simulink model "complex_dbe_core"  (Simulink 7.1)
settings: Solver=ode45  StartTime=0.0  StopTime=1000  RelTol=1e-3
libraries: xbsIndex_r4 x308, cfa_library x64, casper_library_misc x6, simulink x2
(part 1 of 6)
settings Model: Creator=Administrator  LastModifiedBy=Administrator

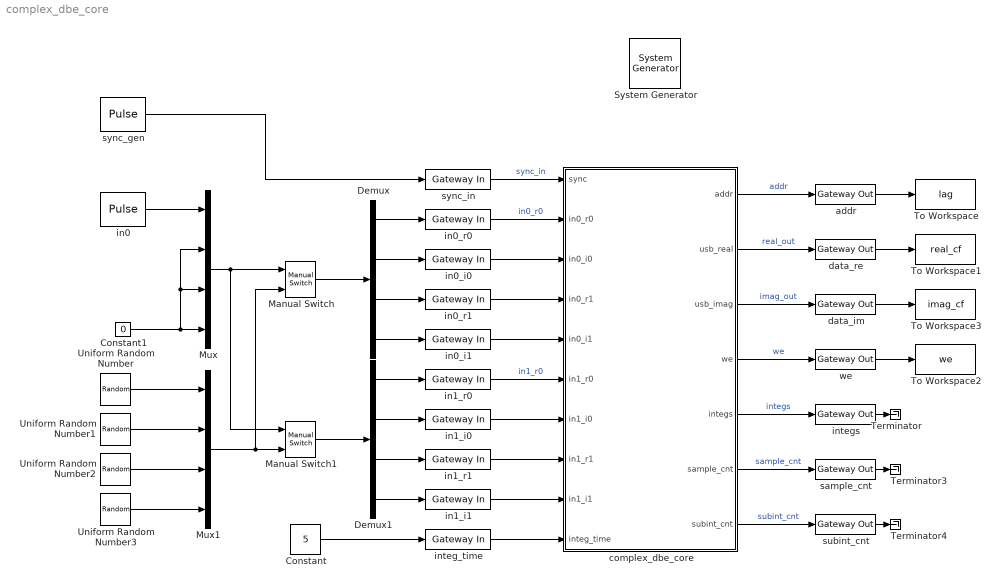
== system complex_dbe_core ==
  " System Generator" : xbsIndex_r4/ System Generator  Tag=genX  SystemSampleTime=-1  xilinxfamily=virtex2p  part=xc2vp50  speed=-7  package=ff1152  synthesis_tool=XST  clock_wrapper=Clock Enables  directory=./complex_dbe_core  testbench=off  simulink_period=1  sysclk_period=10  dcm_input_clock_period=100  incr_netlist=off  trim_vbits=Everywhere in SubSystem  dbl_ovrd=According to Block Masks  core_generation=According to Block Masks  run_coregen=off  deprecated_control=off  eval_field=0  block_type=sysgen
      settings: block_version=10.1.3
  Constant : Constant  Value=5  OutDataType=sfix(16)  OutScaling=2^0
  Constant1 : Constant  Value=0
  Demux : Demux
  Demux1 : Demux
  Manual Switch : simulink/Signal Routing/Manual Switch  SystemSampleTime=-1  sw=0  action=0  varsize=off
  Manual Switch1 : simulink/Signal Routing/Manual Switch  SystemSampleTime=-1  sw=0  action=0  varsize=off
  Mux : Mux
  Mux1 : Mux
  Terminator : Terminator
  Terminator3 : Terminator
  Terminator4 : Terminator
  To Workspace : ToWorkspace  VariableName=lag  SampleTime=-1  SaveFormat=Array
  To Workspace1 : ToWorkspace  VariableName=real_cf  SampleTime=-1  SaveFormat=Array
  To Workspace2 : ToWorkspace  VariableName=we  SampleTime=-1  SaveFormat=Array
  To Workspace3 : ToWorkspace  VariableName=imag_cf  SampleTime=-1  SaveFormat=Array
  Uniform Random Number : UniformRandomNumber  Minimum=0  Maximum=3  Seed=1111  SampleTime=1
  Uniform Random Number1 : UniformRandomNumber  Minimum=0  Maximum=3  Seed=2222  SampleTime=1
  Uniform Random Number2 : UniformRandomNumber  Minimum=0  Maximum=3  Seed=3333  SampleTime=1
  Uniform Random Number3 : UniformRandomNumber  Minimum=0  Maximum=3  Seed=4444  SampleTime=1
  addr : xbsIndex_r4/Gateway Out  hdl_port=on  timing_constraint=None  locs_specified=off  LOCs={}  block_type=gatewayout
      settings: infoedit="Gateway out block.  Converts Xilinx fixed point inputs into ouputs of type Simulink integer, double, or fixed point.<P><P>Hardware notes:  In hardware these blocks become top level output ports or are discarded, depending on how they are configured."  block_version=10.1.3
  complex_dbe_core : Subsystem
  data_im : xbsIndex_r4/Gateway Out  hdl_port=on  timing_constraint=None  locs_specified=off  LOCs={}  block_type=gatewayout
      settings: infoedit="Gateway out block.  Converts Xilinx fixed point inputs into ouputs of type Simulink integer, double, or fixed point.<P><P>Hardware notes:  In hardware these blocks become top level output ports or are discarded, depending on how they are configured."  block_version=10.1.3
  data_re : xbsIndex_r4/Gateway Out  hdl_port=on  timing_constraint=None  locs_specified=off  LOCs={}  block_type=gatewayout
      settings: infoedit="Gateway out block.  Converts Xilinx fixed point inputs into ouputs of type Simulink integer, double, or fixed point.<P><P>Hardware notes:  In hardware these blocks become top level output ports or are discarded, depending on how they are configured."  block_version=10.1.3
  in0 : DiscretePulseGenerator  Period=1e4  PhaseDelay=256+10+1+16*2
      settings: AttributesFormatString=%<PulseWidth> wide\npulse at %<PhaseDelay>\nevery %<Period>
  in0_i0 : xbsIndex_r4/Gateway In  arith_type=Unsigned  n_bits=2  bin_pt=0  quantization=Truncate  overflow=Wrap  period=1  dbl_ovrd=off  timing_constraint=None  locs_specified=off  LOCs={}  block_type=gatewayin
      settings: infoedit="Gateway in block.  Converts inputs of type Simulink integer, double and fixed point to  Xilinx fixed point type.<br><br>Hardware notes:  In hardware these blocks become top level input ports."  block_version=10.1.3
  in0_i1 : xbsIndex_r4/Gateway In  arith_type=Unsigned  n_bits=2  bin_pt=0  quantization=Truncate  overflow=Wrap  period=1  dbl_ovrd=off  timing_constraint=None  locs_specified=off  LOCs={}  block_type=gatewayin
      settings: infoedit="Gateway in block.  Converts inputs of type Simulink integer, double and fixed point to  Xilinx fixed point type.<br><br>Hardware notes:  In hardware these blocks become top level input ports."  block_version=10.1.3
  in0_r0 : xbsIndex_r4/Gateway In  arith_type=Unsigned  n_bits=2  bin_pt=0  quantization=Truncate  overflow=Flag as error  period=1  dbl_ovrd=off  timing_constraint=None  locs_specified=off  LOCs={}  block_type=gatewayin
      settings: infoedit="Gateway in block.  Converts inputs of type Simulink integer, double and fixed point to  Xilinx fixed point type.<br><br>Hardware notes:  In hardware these blocks become top level input ports."  block_version=10.1.3
  in0_r1 : xbsIndex_r4/Gateway In  arith_type=Unsigned  n_bits=2  bin_pt=0  quantization=Truncate  overflow=Wrap  period=1  dbl_ovrd=off  timing_constraint=None  locs_specified=off  LOCs={}  block_type=gatewayin
      settings: infoedit="Gateway in block.  Converts inputs of type Simulink integer, double and fixed point to  Xilinx fixed point type.<br><br>Hardware notes:  In hardware these blocks become top level input ports."  block_version=10.1.3
  in1_i0 : xbsIndex_r4/Gateway In  arith_type=Unsigned  n_bits=2  bin_pt=0  quantization=Truncate  overflow=Wrap  period=1  dbl_ovrd=off  timing_constraint=None  locs_specified=off  LOCs={}  block_type=gatewayin
      settings: infoedit="Gateway in block.  Converts inputs of type Simulink integer, double and fixed point to  Xilinx fixed point type.<br><br>Hardware notes:  In hardware these blocks become top level input ports."  block_version=10.1.3
  in1_i1 : xbsIndex_r4/Gateway In  arith_type=Unsigned  n_bits=2  bin_pt=0  quantization=Truncate  overflow=Wrap  period=1  dbl_ovrd=off  timing_constraint=None  locs_specified=off  LOCs={}  block_type=gatewayin
      settings: infoedit="Gateway in block.  Converts inputs of type Simulink integer, double and fixed point to  Xilinx fixed point type.<br><br>Hardware notes:  In hardware these blocks become top level input ports."  block_version=10.1.3
  in1_r0 : xbsIndex_r4/Gateway In  arith_type=Unsigned  n_bits=2  bin_pt=0  quantization=Truncate  overflow=Wrap  period=1  dbl_ovrd=off  timing_constraint=None  locs_specified=off  LOCs={}  block_type=gatewayin
      settings: infoedit="Gateway in block.  Converts inputs of type Simulink integer, double and fixed point to  Xilinx fixed point type.<br><br>Hardware notes:  In hardware these blocks become top level input ports."  block_version=10.1.3
  in1_r1 : xbsIndex_r4/Gateway In  arith_type=Unsigned  n_bits=2  bin_pt=0  quantization=Truncate  overflow=Wrap  period=1  dbl_ovrd=off  timing_constraint=None  locs_specified=off  LOCs={}  block_type=gatewayin
      settings: infoedit="Gateway in block.  Converts inputs of type Simulink integer, double and fixed point to  Xilinx fixed point type.<br><br>Hardware notes:  In hardware these blocks become top level input ports."  block_version=10.1.3
  integ_time : xbsIndex_r4/Gateway In  arith_type=Unsigned  n_bits=32  bin_pt=0  quantization=Truncate  overflow=Wrap  period=1  dbl_ovrd=off  timing_constraint=None  locs_specified=off  LOCs={}  block_type=gatewayin
      settings: infoedit="Gateway in block.  Converts inputs of type Simulink integer, double and fixed point to  Xilinx fixed point type.<P><P>Hardware notes:  In hardware these blocks become top level input ports."  block_version=10.1.3
  integs : xbsIndex_r4/Gateway Out  hdl_port=on  timing_constraint=None  locs_specified=off  LOCs={}  block_type=gatewayout
      settings: infoedit="Gateway out block.  Converts Xilinx fixed point inputs into ouputs of type Simulink integer, double, or fixed point.<P><P>Hardware notes:  In hardware these blocks become top level output ports or are discarded, depending on how they are configured."  block_version=10.1.3
  sample_cnt : xbsIndex_r4/Gateway Out  hdl_port=on  timing_constraint=None  locs_specified=off  LOCs={}  block_type=gatewayout
      settings: infoedit="Gateway out block.  Converts Xilinx fixed point inputs into ouputs of type Simulink integer, double, or fixed point.<P><P>Hardware notes:  In hardware these blocks become top level output ports or are discarded, depending on how they are configured."  block_version=10.1.3
  subint_cnt : xbsIndex_r4/Gateway Out  hdl_port=on  timing_constraint=None  locs_specified=off  LOCs={}  block_type=gatewayout
      settings: infoedit="Gateway out block.  Converts Xilinx fixed point inputs into ouputs of type Simulink integer, double, or fixed point.<P><P>Hardware notes:  In hardware these blocks become top level output ports or are discarded, depending on how they are configured."  block_version=10.1.3
  sync_gen : DiscretePulseGenerator  Period=32  PhaseDelay=10
      settings: AttributesFormatString=%<PulseWidth> wide\npulse at %<PhaseDelay>\nevery %<Period>
  sync_in : xbsIndex_r4/Gateway In  arith_type=Boolean  n_bits=16  bin_pt=14  quantization="Round  (unbiased: +/- Inf)"  overflow=Saturate  period=1  dbl_ovrd=off  timing_constraint=None  locs_specified=off  LOCs={}  block_type=gatewayin
      settings: infoedit="Gateway in block.  Converts inputs of type Simulink integer, double and fixed point to  Xilinx fixed point type.<P><P>Hardware notes:  In hardware these blocks become top level input ports."  block_version=10.1.3
  we : xbsIndex_r4/Gateway Out  hdl_port=on  timing_constraint=None  locs_specified=off  LOCs={}  block_type=gatewayout
      settings: infoedit="Gateway out block.  Converts Xilinx fixed point inputs into ouputs of type Simulink integer, double, or fixed point.<P><P>Hardware notes:  In hardware these blocks become top level output ports or are discarded, depending on how they are configured."  block_version=10.1.3
  wires:
  sync_in/1 -> complex_dbe_core/1(sync)  "sync_in"
  in0_r0/1 -> complex_dbe_core/2(in0_r0)  "in0_r0"
  in0_i0/1 -> complex_dbe_core/3(in0_i0)
  in0_r1/1 -> complex_dbe_core/4(in0_r1)
  in0_i1/1 -> complex_dbe_core/5(in0_i1)
  in1_r0/1 -> complex_dbe_core/6(in1_r0)  "in1_r0"
  in1_i0/1 -> complex_dbe_core/7(in1_i0)
  in1_r1/1 -> complex_dbe_core/8(in1_r1)
  in1_i1/1 -> complex_dbe_core/9(in1_i1)
  sync_gen/1 -> sync_in/1
  integ_time/1 -> complex_dbe_core/10(integ_time)
  Constant/1 -> integ_time/1
  addr/1 -> To Workspace/1
  data_re/1 -> To Workspace1/1
  we/1 -> To Workspace2/1
  complex_dbe_core/1(addr) -> addr/1  "addr"
  complex_dbe_core/2(usb_real) -> data_re/1  "real_out"
  data_im/1 -> To Workspace3/1
  complex_dbe_core/3(usb_imag) -> data_im/1  "imag_out"
  complex_dbe_core/4(we) -> we/1  "we"
  complex_dbe_core/5(integs) -> integs/1  "integs"
  integs/1 -> Terminator/1
  complex_dbe_core/6(sample_cnt) -> sample_cnt/1  "sample_cnt"
  sample_cnt/1 -> Terminator3/1
  complex_dbe_core/7(subint_cnt) -> subint_cnt/1  "subint_cnt"
  subint_cnt/1 -> Terminator4/1
  Demux/1 -> in0_r0/1
  Demux/2 -> in0_i0/1
  Demux/3 -> in0_r1/1
  Demux/4 -> in0_i1/1
  in0/1 -> Mux/1
  Constant1/1 -> Mux/4, Mux/2, Mux/3
  Demux1/1 -> in1_r0/1
  Demux1/2 -> in1_i0/1
  Demux1/3 -> in1_r1/1
  Demux1/4 -> in1_i1/1
  Uniform Random Number/1 -> Mux1/1
  Uniform Random Number1/1 -> Mux1/2
  Uniform Random Number2/1 -> Mux1/3
  Uniform Random Number3/1 -> Mux1/4
  Manual Switch/1 -> Demux/1
  Mux/1 -> Manual Switch/1, Manual Switch1/1
  Manual Switch1/1 -> Demux1/1
  Mux1/1 -> Manual Switch1/2, Manual Switch/2

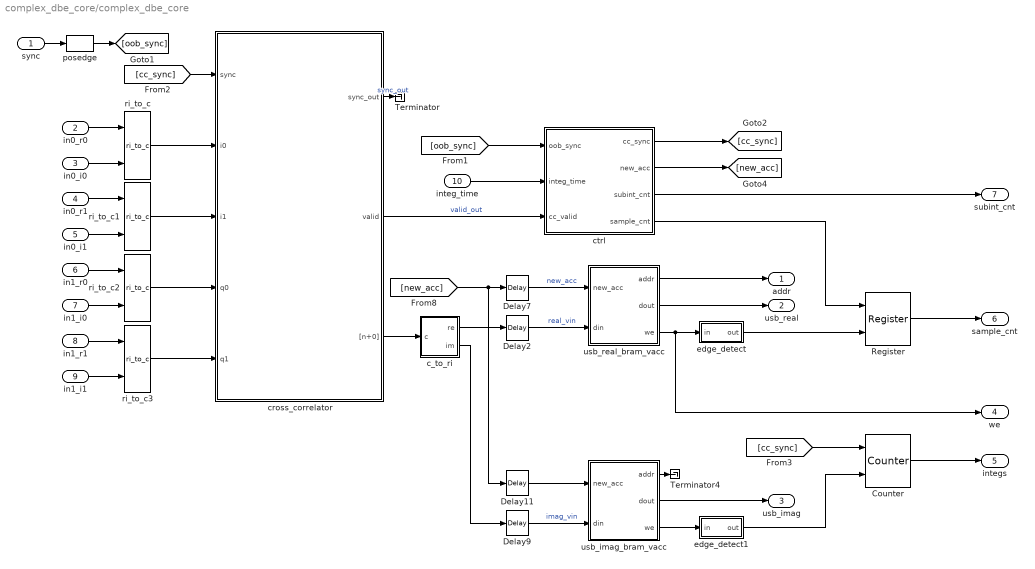
== system complex_dbe_core/complex_dbe_core ==
  sync : Inport
  in0_r0 : Inport  Port=2
  in0_i0 : Inport  Port=3
  in0_r1 : Inport  Port=4
  in0_i1 : Inport  Port=5
  in1_r0 : Inport  Port=6
  in1_i0 : Inport  Port=7
  in1_r1 : Inport  Port=8
  in1_i1 : Inport  Port=9
  integ_time : Inport  Port=10
  Counter : xbsIndex_r4/Counter  cnt_type=Free Running  cnt_to=Inf  operation=Up  start_count=0  cnt_by_val=1  arith_type=Unsigned  n_bits=32  bin_pt=0  load_pin=off  rst=on  en=on  explicit_period=on  period=1  dbl_ovrd=off  use_behavioral_HDL=off  use_rpm=off  implementation=Fabric  block_type=counter
  Delay{2,7,9,11} (4 alike) : xbsIndex_r4/Delay  en=off  latency=1  dbl_ovrd=off  reg_retiming=off  block_type=delay
      settings: block_version=11.4
  Register : xbsIndex_r4/Register  init=0  rst=off  en=on  dbl_ovrd=off  block_type=register
  Terminator : Terminator
  Terminator4 : Terminator
  c_to_ri : Subsystem
  cross_correlator : Subsystem  AncestorBlock=cfa_library/cross_correlator  mask(cross_correlator){total_lags=4, n_inputs=1, use_2bit=on, complex_in=on, input_bit_width=8, input_bin_pt=7, specify_data_type=off, output_bit_width=16, output_bin_pt=14, quantization=Truncate, overflow=Wrap, specify_mult=off, mult_spec=Behavioral, specify_add=off, add_spec=Fabric, mult_delay=3, add_delay=2, overall_delay=1, single_output=on}
      mask prompts: total_lags "Total Lags Centered at Zero: (2^?)"; n_inputs "Number of Simultaneous Inputs: (2^?)"; use_2bit "Use special 2-bit binary encoding"; complex_in "Complex inputs"; input_bit_width "Input Bit Width:"; input_bin_pt "Input Binary Point:"; specify_data_type "Specify output data type"; output_bit_width "Output Bit Width:"; output_bin_pt "Output Binary Point:"; quantization "Quantization Behavior:"; overflow "Overflow Behavior"; specify_mult "Specify multiplier use (behavioural HDL if not specified)"; mult_spec "Multiplier specification:"; specify_add "Specify adder use (behavioural HDL if not specified)"; add_spec "Adder specification:"; mult_delay "Mult Latency:"; add_delay "Add Latency:"; overall_delay "Overall latency:"; single_output "Provide single output stream"
      mask help: This time-domain cross correlator accepts two real time-series and outputs the cross-correlation function for the given set of lags. The output is accumulated so that for every two input samples there is exactly one output sample.
      mask init:
      | cross_correlator_init(gcb,...
      |     'total_lags', total_lags,...
      |     'n_inputs', n_inputs,...
      |     'use_2bit', use_2bit,...
      |     'input_bit_width', input_bit_width,...
      |     'input_bin_pt', input_bin_pt,...
      |     'complex_in', complex_in,...
      |     'specify_data_type', specify_data_type,...
      |     'output_bit_width', output_bit_width,...
      |     'output_bin_pt', output_bin_pt,...
      |     'quantization', quantization,...
      |     'overflow', overflow,...
      |     'specify_mult', specify_mult,...
      |     'mult_spec', mult_spec,...
      |     'specify_add', specify_add,...
      |     'add_spec', add_spec,...
      |     'mult_delay', mult_delay,...
      |     'add_delay', add_delay,...
      |     'overall_delay', overall_delay,...
      |     'single_output', single_output);
      settings: AttributesFormatString=|
      | 16 lags, Demux: 2, Outputs: 1
      | Special 2-bit complex binary encoding
      |  Mult: Behavioral, Add: Fabric
      mask StyleString: edit,edit,checkbox,checkbox,edit,edit,checkbox,edit,edit,popup(Truncate|Round (unbiased: +/- Inf)|Round (unbiased: Even Values)),popup(Wrap|Saturate|Flag as error),checkbox,popup(Behavioral|Core|Embedded),checkbox,popup(Fabric|DSP48),edit,edit,edit,checkbox
      mask CallbackString:
      | ||use_2bit = get_param(gcb,'use_2bit');
      | enables = get_param(gcb, 'MaskEnables');
      | if( strcmp(use_2bit,'on')),
      |     enables{4} = 'on';
      |     enables{5} = 'off';
      |     enables{6} = 'off';
      | else
      |     enables{4} = 'off';
      |     enables{5} = 'on';
      |     enables{6} = 'on';
      |     set_param(gcb, 'complex_in', 'off');
      | end
      | set_param(gcb, 'MaskEnables', enables);
      | ||||specify_data_type = get_param(gcb,'specify_data_type');
      | enables = get_param(gcb, 'MaskEnables');
      | if( strcmp(specify_data_type,'off')),
      |     enables{8} = 'off';
      |     enables{9} = 'off';
      |     enables{10} = 'off';
      |     enables{11} = 'off';
      | else
      |     enables{8} = 'on';
      |     enables{9} = 'on';
      |     enables{10} = 'on';
      |     enables{11} = 'on';
      | end
      | set_param(gcb, 'MaskEnables', enables);
      | |||||specify_mult = get_param(gcb,'specify_mult');
      | enables = get_param(gcb, 'MaskEnables');
      | if( strcmp(specify_mult,'off')),
      |     enables{13} = 'off';
      | else
      |     enables{13} = 'on';
      | end
      | set_param(gcb, 'MaskEnables', enables);
      | ||specify_add = get_param(gcb,'specify_add');
      | enables = get_param(gcb, 'MaskEnables');
      | if( strcmp(specify_add,'off')),
      |     enables{15} = 'off';
      | else
      |     enables{15} = 'on';
      | end
      | set_param(gcb, 'MaskEnables', enables);
      | |||||
      mask TabNameString: Basic,Basic,Input,Input,Input,Input,Output,Output,Output,Output,Output,Implementation,Implementation,Implementation,Implementation,Implementation,Implementation,Implementation,Basic
  ctrl : Subsystem
  edge_detect : Subsystem  AncestorBlock=casper_library_misc/edge_detect  mask(edge_detect){edge=Falling, polarity=Active High, x_in=[0 0.08 0.08 0.16 0.16 0.24 0.24 0.32 0.32 0.4], y_in=[1  1 -1 -1 -1 -1 -1 -1 -1 -1], x_out=[0.6 0.68 0.68 0.76 0.76 0.84 0.84 0.92 0.92 1], y_out=[-1 -1  1  1 -1 -1 -1 -1 -1 -1]}
      mask prompts: edge "Edge Type"; polarity "Output Polarity"; x_in "Input X Positions"; y_in "Input Y Positions"; x_out "Output X Positions"; y_out "Output Y Positions"
      mask help: Output is active for one-cycle after each edge of the specified type (i.e. rising, falling or both).
      mask init:
      | edge_detect_init(gcb,...
      |     'edge',edge,...
      |     'polarity',polarity,...
      |     'x_in',x_in,...
      |     'x_out',x_out,...
      |     'y_in',y_in,...
      |     'y_out',y_out);
      | 
      | x_in_num=str2num(getfield(getfield(get_param(gcb,'UserData'),'parameters'),'x_in'));
      | x_out_num=str2num(getfield(getfield(get_param(gcb,'UserData'),'parameters'),'x_out'));
      | y_in_num=str2num(getfield(getfield(get_param(gcb,'UserData'),'parameters'),'y_in'));
      | y_out_num=str2num(getfield(getfield(get_param(gcb,'UserData'),'parameters'),'y_out'));
      settings: AttributesFormatString=|
      | falling edges
      | active high
      mask Help: Output is active for one-cycle after each edge of the specified type (i.e. rising, falling, or both).  Latency is zero.
      mask StyleString: popup(Rising|Falling|Both),popup(Active High|Active Low),edit,edit,edit,edit
      mask Display:
      | plot(x_in_num,0.5+y_in_num*0.2);
      | plot(x_out_num,0.5+y_out_num*0.2);
  edge_detect1 : Subsystem  AncestorBlock=casper_library_misc/edge_detect  mask(edge_detect){edge=Falling, polarity=Active High, x_in=[0 0.08 0.08 0.16 0.16 0.24 0.24 0.32 0.32 0.4], y_in=[1  1 -1 -1 -1 -1 -1 -1 -1 -1], x_out=[0.6 0.68 0.68 0.76 0.76 0.84 0.84 0.92 0.92 1], y_out=[-1 -1  1  1 -1 -1 -1 -1 -1 -1]}
      mask prompts: edge "Edge Type"; polarity "Output Polarity"; x_in "Input X Positions"; y_in "Input Y Positions"; x_out "Output X Positions"; y_out "Output Y Positions"
      mask help: Output is active for one-cycle after each edge of the specified type (i.e. rising, falling or both).
      mask init: same as complex_dbe_core/complex_dbe_core/edge_detect
      settings: AttributesFormatString=|
      | falling edges
      | active high
      mask Help: Output is active for one-cycle after each edge of the specified type (i.e. rising, falling, or both).  Latency is zero.
      mask StyleString: popup(Rising|Falling|Both),popup(Active High|Active Low),edit,edit,edit,edit
      mask Display:
      | plot(x_in_num,0.5+y_in_num*0.2);
      | plot(x_out_num,0.5+y_out_num*0.2);
  posedge : casper_library_misc/posedge  Tag=Rising Edge Detector  SystemSampleTime=-1
  ri_to_c{,1..3} (4 alike) : casper_library_misc/ri_to_c  SystemSampleTime=-1
  usb_imag_bram_vacc : Subsystem
  usb_real_bram_vacc : Subsystem
  addr : Outport
  usb_real : Outport  Port=2
  usb_imag : Outport  Port=3
  we : Outport  Port=4
  integs : Outport  Port=5
  sample_cnt : Outport  Port=6
  subint_cnt : Outport  Port=7
  wires:
  Delay2/1 -> usb_real_bram_vacc/2(din)  "real_vin"
  [new_acc] -> Delay7/1, Delay11/1
  usb_real_bram_vacc/2(dout) -> usb_real/1
  sync/1 -> posedge/1
  usb_real_bram_vacc/3(we) -> edge_detect/1(in), we/1
  posedge/1 -> [oob_sync]
  cross_correlator/2(valid) -> ctrl/3(cc_valid)  "valid_out"
  [cc_sync] -> cross_correlator/1(sync)
  Delay7/1 -> usb_real_bram_vacc/1(new_acc)  "new_acc"
  ri_to_c2/1 -> cross_correlator/4(q0)
  ri_to_c3/1 -> cross_correlator/5(q1)
  c_to_ri/1(re) -> Delay2/1
  cross_correlator/3("[n+0]") -> c_to_ri/1(c)
  Delay9/1 -> usb_imag_bram_vacc/2(din)  "imag_vin"
  usb_imag_bram_vacc/2(dout) -> usb_imag/1
  Delay11/1 -> usb_imag_bram_vacc/1(new_acc)
  c_to_ri/2(im) -> Delay9/1
  ri_to_c/1 -> cross_correlator/2(i0)
  ri_to_c1/1 -> cross_correlator/3(i1)
  in0_r0/1 -> ri_to_c/1
  in0_i0/1 -> ri_to_c/2
  in0_r1/1 -> ri_to_c1/1
  in0_i1/1 -> ri_to_c1/2
  in1_r0/1 -> ri_to_c2/1
  in1_i0/1 -> ri_to_c2/2
  in1_r1/1 -> ri_to_c3/1
  in1_i1/1 -> ri_to_c3/2
  usb_imag_bram_vacc/3(we) -> edge_detect1/1(in)
  ctrl/1(cc_sync) -> [cc_sync]
  ctrl/2(new_acc) -> [new_acc]
  integ_time/1 -> ctrl/2(integ_time)
  [oob_sync] -> ctrl/1(oob_sync)
  usb_real_bram_vacc/1(addr) -> addr/1
  ctrl/4(sample_cnt) -> Register/1
  edge_detect/1(out) -> Register/2
  ctrl/3(subint_cnt) -> subint_cnt/1
  edge_detect1/1(out) -> Counter/2
  Register/1 -> sample_cnt/1
  Counter/1 -> integs/1
  [cc_sync] -> Counter/1
  cross_correlator/1(sync_out) -> Terminator/1  "sync_out"
  usb_imag_bram_vacc/1(addr) -> Terminator4/1

== system complex_dbe_core/complex_dbe_core/c_to_ri ==
  c : Inport
  BitBasher : xbsIndex_r4/BitBasher  bitexpr=|  display_expr=off  sr_1=1  arith_type1="Signed  (2's comp)"  bin_pt1=0  sr_2=2  arith_type2="Signed  (2's comp)"  bin_pt2=0  sr_3=3  arith_type3=Unsigned  bin_pt3=0  sr_4=4  arith_type4=Unsigned  bin_pt4=0  dbl_ovrd=off  block_type=bitbasher
      | <html><head><meta name="qrichtext" content="1" /><style type="text/css">
      | p, li { white-space: pre-wrap; }
      | </style></head><body style=" font-family:'MS Shell Dlg 2'; font-size:8.25pt; font-weight:400; font-style:normal;">
      | <p style=" margin-top:12px; margin-bottom:12px; margin-left:0px; margin-right:0px; -qt-block-indent:0; text-indent:0px; font-family:'MS Shell Dlg'; font-size:8pt;">re={c[21:12]}<br />im={c[10:1]}</p></body></html>
      settings: block_version=10.1.3
  re : Outport
  im : Outport  Port=2
  wires:
  BitBasher/1 -> re/1
  c/1 -> BitBasher/1
  BitBasher/2 -> im/1
